simulink model "SPO10_simplified"  (R2018b)
settings: Solver=FixedStepAuto  StartTime=0.0  StopTime=inf  RelTol=1e-3
values from neighbouring files (symbols this model uses):
  az = (-180:180)    [init.m]
  az_H_B = interp1(f_B.az_E_phi(~isnan(f_B.az_E_phi)), f_B.az_E_r(~isnan(f_B.az_E_r)), az, 'pchip', 0)    [init.m]
  az_V_B = interp1(f_B.el_H_phi(~isnan(f_B.el_H_phi)), f_B.el_H_r(~isnan(f_B.el_H_r)), az, 'pchip', 0)    [init.m]
undefined symbols (not defined in the file or in its folder): Busy, Wait
libraries: simulink x9, powerlib_meascontrol x4, aerolibanimutils x1
settings Model: Creator=matib  LastModifiedBy=matib

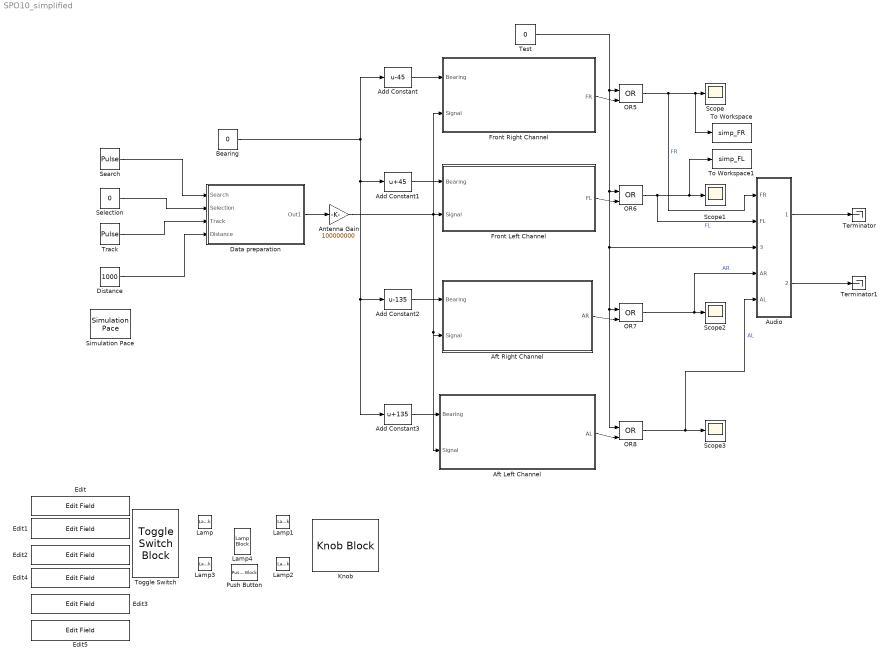
== system SPO10_simplified ==
  Add Constant : Bias  Bias=-45
  Add Constant1 : Bias  Bias=45
  Add Constant2 : Bias  Bias=-135
  Add Constant3 : Bias  Bias=135
  Aft Left Channel : Subsystem
  Aft Right Channel : Subsystem
  Antenna Gain : Gain  Gain=100000000
  Audio : Subsystem
  Bearing : Constant  Value=0
  Data preparation : Subsystem
  Distance : Constant  Value=1000
  Edit : EditField  WebBlockId=126  LabelPosition=Bottom  ShowInitialText=on  Alignment=Center
  Edit1 : EditField  WebBlockId=127  LabelPosition=Bottom  ShowInitialText=on  Alignment=Center
  Edit2 : EditField  WebBlockId=128  LabelPosition=Bottom  ShowInitialText=on  Alignment=Center
  Edit3 : EditField  WebBlockId=129  LabelPosition=Bottom  ShowInitialText=on  Alignment=Center
  Edit4 : EditField  WebBlockId=130  LabelPosition=Bottom  ShowInitialText=on  Alignment=Center
  Edit5 : EditField  WebBlockId=131  LabelPosition=Bottom  ShowInitialText=on  Alignment=Center
  Front Left Channel : Subsystem
  Front Right Channel : Subsystem
  Knob : KnobBlock  WebBlockId=97  LabelPosition=Bottom  ScaleMax=1
  Lamp : LampBlock  WebBlockId=86  LabelPosition=Hide
  Lamp1 : LampBlock  WebBlockId=90  LabelPosition=Hide
  Lamp2 : LampBlock  WebBlockId=91  LabelPosition=Hide
  Lamp3 : LampBlock  WebBlockId=92  LabelPosition=Hide
  Lamp4 : LampBlock  WebBlockId=96
  OR{5..8} (4 alike) : Logic  Operator=OR  IconShape=distinctive  AllPortsSameDT=off  OutDataTypeStr=boolean
  Push Button : PushButtonBlock  WebBlockId=105  ButtonText=Test
  Scope{,1..3} (4 alike) : Scope
  Search : DiscretePulseGenerator  PulseType=Time based  Period=1  PulseWidth=1/60*100
  Selection : Constant  Value=0
  Simulation Pace : aerolibanimutils/Simulation Pace  SimulationPace=1  SleepMode=Busy-Wait  OutputPaceError=off  SampleTime=-1
  Terminator : Terminator
  Terminator1 : Terminator
  Test : Constant  Value=0
  To Workspace : ToWorkspace  VariableName=simp_FR  SaveFormat=Timeseries  SampleTime=-1
  To Workspace1 : ToWorkspace  VariableName=simp_FL  SaveFormat=Timeseries  SampleTime=-1
  Toggle Switch : ToggleSwitchBlock  WebBlockId=11  LabelPosition=Hide
      settings: Values={{'Track', 'Search'}, [0 1]}
  Track : DiscretePulseGenerator  PulseType=Time based  Period=1/60  PulseWidth=50
  wires:
  Antenna Gain/1 -> Front Left Channel/2(Signal), Front Right Channel/2(Signal), Aft Left Channel/2(Signal), Aft Right Channel/2(Signal)
  Bearing/1 -> Add Constant3/1, Add Constant2/1, Add Constant1/1, Add Constant/1
  OR5/1 -> Audio/1(FR), To Workspace/1, Scope/1  "FR"
  OR6/1 -> Audio/2(FL), To Workspace1/1, Scope1/1  "FL"
  OR7/1 -> Audio/4(AR), Scope2/1  "AR"
  OR8/1 -> Audio/5(AL), Scope3/1  "AL"
  Test/1 -> OR8/1, OR7/1, Audio/3(Test), OR6/1, OR5/1
  Search/1 -> Data preparation/1(Search)
  Selection/1 -> Data preparation/2(Selection)
  Track/1 -> Data preparation/3(Track)
  Distance/1 -> Data preparation/4(Distance)
  Data preparation/1(Out1) -> Antenna Gain/1
  Add Constant/1 -> Front Right Channel/1(Bearing)
  Front Right Channel/1(FR) -> OR5/2
  Add Constant1/1 -> Front Left Channel/1(Bearing)
  Front Left Channel/1(FL) -> OR6/2
  Add Constant2/1 -> Aft Right Channel/1(Bearing)
  Aft Right Channel/1(AR) -> OR7/2
  Add Constant3/1 -> Aft Left Channel/1(Bearing)
  Aft Left Channel/1(AL) -> OR8/2
  Audio/1(No sound) -> Terminator/1
  Audio/2(Audo out) -> Terminator1/1

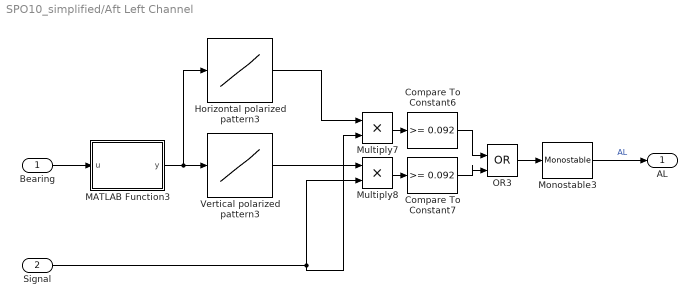
== system SPO10_simplified/Aft Left Channel ==
  Bearing : Inport
  Signal : Inport  Port=2
  Compare To Constant6 : simulink/Logic and Bit Operations/Compare To Constant  relop=>=  const=0.092  OutDataTypeStr=boolean
  Compare To Constant7 : simulink/Logic and Bit Operations/Compare To Constant  relop=>=  const=0.092  OutDataTypeStr=boolean
  Horizontal polarized pattern3 : Lookup_n-D  NumberOfTableDimensions=1  BreakpointsForDimension1=az  BreakpointsForDimension1Min=[-180]  BreakpointsForDimension1Max=[180]  Table=az_H_B  TableMin=[0]  ExtrapMethod=Clip  DiagnosticForOutOfRangeInput=Warning  UseLastTableValue=on  InternalRulePriority=Speed  OutMin=[0]  RndMeth=Simplest  InputSameDT=on
  MATLAB Function3 : MATLAB Function  TreatAsAtomicUnit=on
  Monostable3 : powerlib_meascontrol/Logic/Monostable  EdgeDetect=Rising  PulseDuration=0.08  ic=0  Ts=1/200
      settings: SourceProductName=Simscape Power Systems  SourceProductBaseCode=PS
  Multiply7 : Product
  Multiply8 : Product
  OR3 : Logic  Operator=OR  IconShape=distinctive  AllPortsSameDT=off  OutDataTypeStr=boolean
  Vertical polarized pattern3 : Lookup_n-D  NumberOfTableDimensions=1  BreakpointsForDimension1=az  BreakpointsForDimension1Min=[-180]  BreakpointsForDimension1Max=[180]  Table=az_V_B  TableMin=[0]  ExtrapMethod=Clip  DiagnosticForOutOfRangeInput=Warning  UseLastTableValue=on  InternalRulePriority=Speed  OutMin=[0]  RndMeth=Simplest  InputSameDT=on
  AL : Outport
  wires:
  Horizontal polarized pattern3/1 -> Multiply7/1
  Signal/1 -> Multiply8/2, Multiply7/2
  MATLAB Function3/1(y) -> Horizontal polarized pattern3/1, Vertical polarized pattern3/1
  OR3/1 -> Monostable3/1
  Vertical polarized pattern3/1 -> Multiply8/1
  Multiply7/1 -> Compare To Constant6/1
  Multiply8/1 -> Compare To Constant7/1
  Compare To Constant6/1 -> OR3/1
  Compare To Constant7/1 -> OR3/2
  Bearing/1 -> MATLAB Function3/1(u)
  Monostable3/1 -> AL/1  "AL"

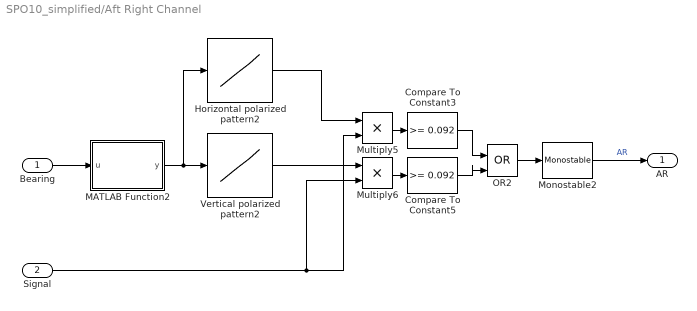
== system SPO10_simplified/Aft Right Channel ==
  Bearing : Inport
  Signal : Inport  Port=2
  Compare To Constant3 : simulink/Logic and Bit Operations/Compare To Constant  relop=>=  const=0.092  OutDataTypeStr=boolean
  Compare To Constant5 : simulink/Logic and Bit Operations/Compare To Constant  relop=>=  const=0.092  OutDataTypeStr=boolean
  Horizontal polarized pattern2 : Lookup_n-D  NumberOfTableDimensions=1  BreakpointsForDimension1=az  BreakpointsForDimension1Min=[-180]  BreakpointsForDimension1Max=[180]  Table=az_H_B  TableMin=[0]  ExtrapMethod=Clip  DiagnosticForOutOfRangeInput=Warning  UseLastTableValue=on  InternalRulePriority=Speed  OutMin=[0]  RndMeth=Simplest  InputSameDT=on
  MATLAB Function2 : MATLAB Function  TreatAsAtomicUnit=on
  Monostable2 : powerlib_meascontrol/Logic/Monostable  EdgeDetect=Rising  PulseDuration=0.08  ic=0  Ts=1/200
      settings: SourceProductName=Simscape Power Systems  SourceProductBaseCode=PS
  Multiply5 : Product
  Multiply6 : Product
  OR2 : Logic  Operator=OR  IconShape=distinctive  AllPortsSameDT=off  OutDataTypeStr=boolean
  Vertical polarized pattern2 : Lookup_n-D  NumberOfTableDimensions=1  BreakpointsForDimension1=az  BreakpointsForDimension1Min=[-180]  BreakpointsForDimension1Max=[180]  Table=az_V_B  TableMin=[0]  ExtrapMethod=Clip  DiagnosticForOutOfRangeInput=Warning  UseLastTableValue=on  InternalRulePriority=Speed  OutMin=[0]  RndMeth=Simplest  InputSameDT=on
  AR : Outport
  wires:
  Multiply6/1 -> Compare To Constant5/1
  MATLAB Function2/1(y) -> Vertical polarized pattern2/1, Horizontal polarized pattern2/1
  Multiply5/1 -> Compare To Constant3/1
  Signal/1 -> Multiply6/2, Multiply5/2
  Monostable2/1 -> AR/1  "AR"
  Compare To Constant3/1 -> OR2/1
  Horizontal polarized pattern2/1 -> Multiply5/1
  OR2/1 -> Monostable2/1
  Compare To Constant5/1 -> OR2/2
  Vertical polarized pattern2/1 -> Multiply6/1
  Bearing/1 -> MATLAB Function2/1(u)

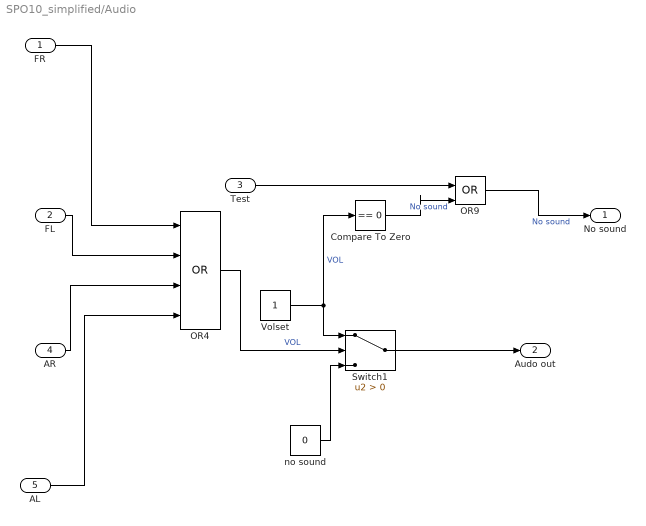
== system SPO10_simplified/Audio ==
  FR : Inport
  FL : Inport  Port=2
  Test : Inport  Port=3
  AR : Inport  Port=4
  AL : Inport  Port=5
  Compare To Zero : simulink/Logic and Bit Operations/Compare To Zero  relop===  OutDataTypeStr=boolean
  OR4 : Logic  Operator=OR  Inputs=4  IconShape=distinctive  AllPortsSameDT=off  OutDataTypeStr=boolean
  OR9 : Logic  Operator=OR  IconShape=distinctive  AllPortsSameDT=off  OutDataTypeStr=boolean
  Switch1 : Switch  Criteria=u2 > Threshold
  Volset : Constant
  no sound : Constant  Value=0
  No sound : Outport
  Audo out : Outport  Port=2
  wires:
  Volset/1 -> Switch1/1, Compare To Zero/1  "VOL"
  OR4/1 -> Switch1/2  "VOL"
  AR/1 -> OR4/3
  FL/1 -> OR4/2
  FR/1 -> OR4/1
  no sound/1 -> Switch1/3
  Compare To Zero/1 -> OR9/2  "No sound"
  Switch1/1 -> Audo out/1
  Test/1 -> OR9/1
  OR9/1 -> No sound/1  "No sound"
  AL/1 -> OR4/4

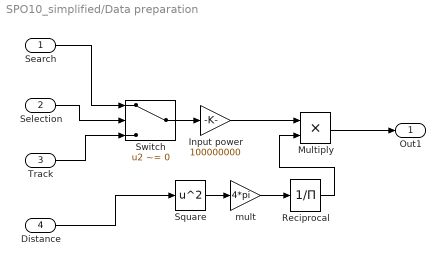
== system SPO10_simplified/Data preparation ==
  Search : Inport
  Selection : Inport  Port=2
  Track : Inport  Port=3
  Distance : Inport  Port=4
  Input power : Gain  Gain=100000000
  Multiply : Product
  Reciprocal : Product  Inputs=/
  Square : Math  Operator=square  SaturateOnIntegerOverflow=on
  Switch : Switch  Criteria=u2 ~= 0
  mult : Gain  Gain=4*pi
  Out1 : Outport
  wires:
  mult/1 -> Reciprocal/1
  Track/1 -> Switch/3
  Selection/1 -> Switch/2
  Input power/1 -> Multiply/1
  Search/1 -> Switch/1
  Reciprocal/1 -> Multiply/2
  Distance/1 -> Square/1
  Square/1 -> mult/1
  Switch/1 -> Input power/1
  Multiply/1 -> Out1/1

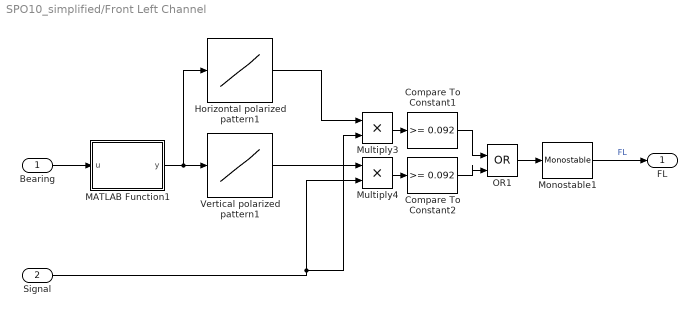
== system SPO10_simplified/Front Left Channel ==
  Bearing : Inport
  Signal : Inport  Port=2
  Compare To Constant1 : simulink/Logic and Bit Operations/Compare To Constant  relop=>=  const=0.092  OutDataTypeStr=boolean
  Compare To Constant2 : simulink/Logic and Bit Operations/Compare To Constant  relop=>=  const=0.092  OutDataTypeStr=boolean
  Horizontal polarized pattern1 : Lookup_n-D  NumberOfTableDimensions=1  BreakpointsForDimension1=az  BreakpointsForDimension1Min=[-180]  BreakpointsForDimension1Max=[180]  Table=az_H_B  TableMin=[0]  ExtrapMethod=Clip  DiagnosticForOutOfRangeInput=Warning  UseLastTableValue=on  InternalRulePriority=Speed  OutMin=[0]  RndMeth=Simplest  InputSameDT=on
  MATLAB Function1 : MATLAB Function  TreatAsAtomicUnit=on
  Monostable1 : powerlib_meascontrol/Logic/Monostable  EdgeDetect=Rising  PulseDuration=0.08  ic=0  Ts=1/200
      settings: SourceProductName=Simscape Power Systems  SourceProductBaseCode=PS
  Multiply3 : Product
  Multiply4 : Product
  OR1 : Logic  Operator=OR  IconShape=distinctive  AllPortsSameDT=off  OutDataTypeStr=boolean
  Vertical polarized pattern1 : Lookup_n-D  NumberOfTableDimensions=1  BreakpointsForDimension1=az  BreakpointsForDimension1Min=[-180]  BreakpointsForDimension1Max=[180]  Table=az_V_B  TableMin=[0]  ExtrapMethod=Clip  DiagnosticForOutOfRangeInput=Warning  UseLastTableValue=on  InternalRulePriority=Speed  OutMin=[0]  RndMeth=Simplest  InputSameDT=on
  FL : Outport
  wires:
  Vertical polarized pattern1/1 -> Multiply4/1
  OR1/1 -> Monostable1/1
  Multiply3/1 -> Compare To Constant1/1
  Signal/1 -> Multiply3/2, Multiply4/2
  MATLAB Function1/1(y) -> Horizontal polarized pattern1/1, Vertical polarized pattern1/1
  Compare To Constant1/1 -> OR1/1
  Multiply4/1 -> Compare To Constant2/1
  Compare To Constant2/1 -> OR1/2
  Monostable1/1 -> FL/1  "FL"
  Bearing/1 -> MATLAB Function1/1(u)
  Horizontal polarized pattern1/1 -> Multiply3/1

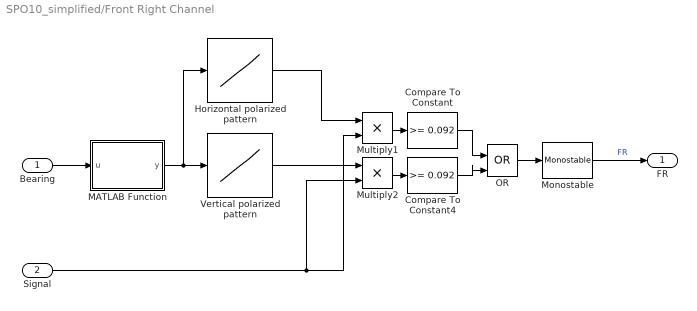
== system SPO10_simplified/Front Right Channel ==
  Bearing : Inport
  Signal : Inport  Port=2
  Compare To Constant : simulink/Logic and Bit Operations/Compare To Constant  relop=>=  const=0.092  OutDataTypeStr=boolean
  Compare To Constant4 : simulink/Logic and Bit Operations/Compare To Constant  relop=>=  const=0.092  OutDataTypeStr=boolean
  Horizontal polarized pattern : Lookup_n-D  NumberOfTableDimensions=1  BreakpointsForDimension1=az  BreakpointsForDimension1Min=[-180]  BreakpointsForDimension1Max=[180]  Table=az_H_B  TableMin=[0]  ExtrapMethod=Clip  DiagnosticForOutOfRangeInput=Warning  UseLastTableValue=on  InternalRulePriority=Speed  OutMin=[0]  RndMeth=Simplest  InputSameDT=on
  MATLAB Function : MATLAB Function  TreatAsAtomicUnit=on
  Monostable : powerlib_meascontrol/Logic/Monostable  EdgeDetect=Rising  PulseDuration=0.08  ic=0  Ts=1/200
      settings: SourceProductName=Simscape Power Systems  SourceProductBaseCode=PS
  Multiply1 : Product
  Multiply2 : Product
  OR : Logic  Operator=OR  IconShape=distinctive  AllPortsSameDT=off  OutDataTypeStr=boolean
  Vertical polarized pattern : Lookup_n-D  NumberOfTableDimensions=1  BreakpointsForDimension1=az  BreakpointsForDimension1Min=[-180]  BreakpointsForDimension1Max=[180]  Table=az_V_B  TableMin=[0]  ExtrapMethod=Clip  DiagnosticForOutOfRangeInput=Warning  UseLastTableValue=on  InternalRulePriority=Speed  OutMin=[0]  RndMeth=Simplest  InputSameDT=on
  FR : Outport
  wires:
  Multiply1/1 -> Compare To Constant/1
  Monostable/1 -> FR/1  "FR"
  Compare To Constant4/1 -> OR/2
  MATLAB Function/1(y) -> Vertical polarized pattern/1, Horizontal polarized pattern/1
  Compare To Constant/1 -> OR/1
  Vertical polarized pattern/1 -> Multiply2/1
  Signal/1 -> Multiply2/2, Multiply1/2
  Multiply2/1 -> Compare To Constant4/1
  OR/1 -> Monostable/1
  Horizontal polarized pattern/1 -> Multiply1/1
  Bearing/1 -> MATLAB Function/1(u)

== matlab function SPO10_simplified/Front Left Channel/MATLAB Function1 ==
  data: u input; y output
function y = clip(u)

    if u<-180
        y=u+360;
    elseif u>180
        y=u-360;
    else
        y=u;
    end

end

== matlab function SPO10_simplified/Front Right Channel/MATLAB Function ==
  data: u input; y output
function y = clip(u)

    if u<-180
        y=u+360;
    elseif u>180
        y=u-360;
    else
        y=u;
    end

end

== matlab function SPO10_simplified/Aft Right Channel/MATLAB Function2 ==
  data: u input; y output
function y = clip(u)

    if u<-180
        y=u+360;
    elseif u>180
        y=u-360;
    else
        y=u;
    end

end

== matlab function SPO10_simplified/Aft Left Channel/MATLAB Function3 ==
  data: u input; y output
function y = clip(u)

    if u<-180
        y=u+360;
    elseif u>180
        y=u-360;
    else
        y=u;
    end

end
